simulink model "DragBlock_V2"  (R2022a)
settings: Solver=VariableStepAuto  StartTime=0.0  StopTime=10.0  RelTol=1e-3
settings Model: Creator=antonisioannou  LastModifiedBy=antonisioannou

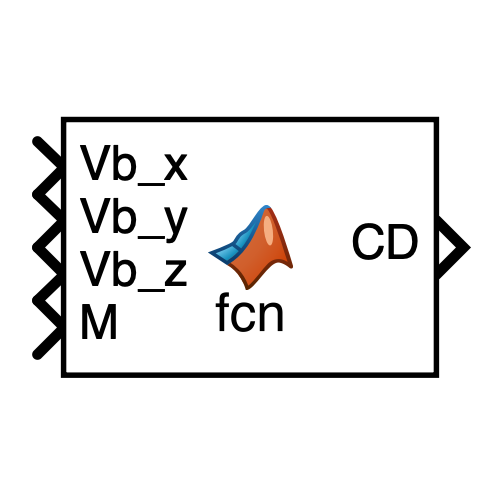
[thumbnail: Simulink's stored preview of the top-level diagram]
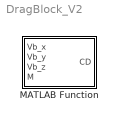
== system DragBlock_V2 ==
  MATLAB Function : MATLAB Function  TreatAsAtomicUnit=on

== matlab function DragBlock_V2/MATLAB Function ==
  data: Vb_x input; Vb_y input; Vb_z input; M input; CD output
function CD = fcn( Vb_x, Vb_y, Vb_z,M)
% funnction takes as inputs Mach number and all velocities on vector form 

% Dimensions

L=   ;  % body legth 
b= ; %Distance from fin-tip to fin-tip
d= ; %Body diameters
f=   ; %Finess ratio
N_f= ; % Number of fins
C_R= ;   %Root fin chord
S_f=C_R*N_F*(b-d)/2 %Fin Surface Area 
Rs=     ;  % surface roughness
Aref=   ;  % surface area
Awet_can= ;% canards wetted are
Awet_fin= ; % fin wetted area 
cbar_fins= s% Cf calculation
d1=  ;     % diameter at the beginning of boattail 
d2= ;      % diameter at the end of the boattail (end of the rocket)
Abase=    %Area at the end of the rocket 
Aboat=     %Area at the start of the boattail
gamma=1/(d1-d2) ; % factor definning boattail profile 
Fin_thetaLE= ;   % Fin leading edge angle 
if Re < 10E04
    Cf=1.48*10^-2;

elseif (10^3<Re) && (Re<Rcrit) 
Cf=1/(1.5*ln(Re)-5.6)^2;

else 
    Cf=0.032*(Rs/L)^0.2;

end

% Cf comdepress. corrwedwedection
Cf=Cf*(1-0.1*M^2);

% CD  due to skin friction of body calc.
CDbody=Cf*((1+1/(2*f))*Awet_body+(1+2*t_f/cbar_fins)*Awet_fins + (1+2*t_c/cbar_can)*Awet_can)/Aref

%  pressure drag 
CDbase=0.12+0.13*M^2; % due to base drag

% The following are for calculating the pressure drag, due to the boattail
if gamma<1
    factor=1;
elseif (1<gamma) && (gamma<3)
factor=(3-gamma)/3;
elseif gamma>3
    factor=0;
end
CD_boat=Abase/Aboat*CDbase*factor; %boattail press. drag 

% Fin pressure drag 
CDfin=((1-M^2)^(-0.417)-1)*(cos(Fin_thetaLE))^2; % For M<0.9
